simulink model "classification_model_1"  (R2018b)
settings: Solver=daessc  StartTime=0.0  StopTime=1  RelTol=1e-3
libraries: powerlib x7, powerlib_meascontrol x2
settings Model: Creator=Edagotti Pavankumar  LastModifiedBy=Edagotti Pavankumar
settings SolverCC: ZeroCrossAlgorithm=Adaptive
settings DebuggingCC: IgnoredZcDiagnostic=none

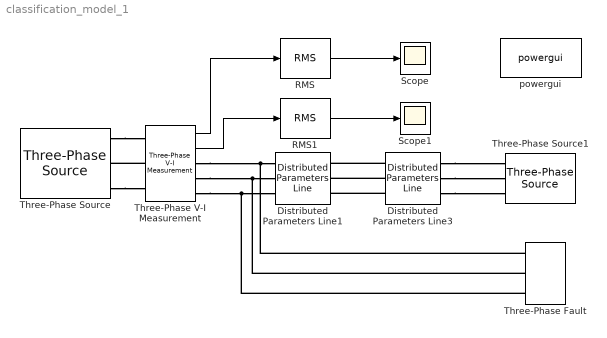
== system classification_model_1 ==
  Distributed Parameters Line1 : powerlib/Elements/Distributed Parameters Line  Phases=3  Frequency=50  Resistance=[0.0238 0.3885]  Inductance=[0.0009509508 0.0032508989]  Capacitance=[12.74e-9 7.751e-9]  Length=50  x1=[2.03029205726985e-09 272935.130000171 272935.130000166;314.159265358979 314.159265358979 314.159265358979;-1.05771318215586 0.434584098775176 -1.13621222801972]  x2=[2.17628988513287e-09 274142.447000751 274142.447000746;314.159265358979 314.159265358979 314.159265358979;-1.04287975057277 0.434398876325849 -1.13639745046905]  x3=[5.79526815658465e-12 1012.46010166729 1012.46010166727;314.159265358979 314.159265358979 314.159265358979;-1.58211710677278 0.326179290986126 -1.24461703580876]  x4=[8.43304661848584e-13 1012.22505654136 1012.22505654134;314.159265358979 314.159265358979 314.159265358979;-1.72619955217939 0.488614155737012 -1.08218217105788]  x5=0.000282770783497871  V1=[2.03e-09 2.729e+05 2.729e+05;314.2 314.2 314.2;-1.058 0.4346 -1.136]  V2=[2.176e-09 2.741e+05 2.741e+05;314.2 314.2 314.2;-1.043 0.4344 -1.136]  I1=[5.795e-12 1012 1012;314.2 314.2 314.2;-1.582 0.3262 -1.245]  I2=[8.433e-13 1012 1012;314.2 314.2 314.2;-1.726 0.4886 -1.082]  nHarmo=1  Measurements=None
      settings: SourceProductName=Simscape Power Systems
  Distributed Parameters Line3 : powerlib/Elements/Distributed Parameters Line  Phases=3  Frequency=50  Resistance=[0.0238 0.3885]  Inductance=[0.0009509508 0.0032508989]  Capacitance=[12.74e-9 7.751e-9]  Length=50  x1=[2.03029205726985e-09 272935.130000171 272935.130000166;314.159265358979 314.159265358979 314.159265358979;-1.05771318215586 0.434584098775176 -1.13621222801972]  x2=[2.17628988513287e-09 274142.447000751 274142.447000746;314.159265358979 314.159265358979 314.159265358979;-1.04287975057277 0.434398876325849 -1.13639745046905]  x3=[5.79526815658465e-12 1012.46010166729 1012.46010166727;314.159265358979 314.159265358979 314.159265358979;-1.58211710677278 0.326179290986126 -1.24461703580876]  x4=[8.43304661848584e-13 1012.22505654136 1012.22505654134;314.159265358979 314.159265358979 314.159265358979;-1.72619955217939 0.488614155737012 -1.08218217105788]  x5=0.000282770783497871  V1=[2.03e-09 2.729e+05 2.729e+05;314.2 314.2 314.2;-1.058 0.4346 -1.136]  V2=[2.176e-09 2.741e+05 2.741e+05;314.2 314.2 314.2;-1.043 0.4344 -1.136]  I1=[5.795e-12 1012 1012;314.2 314.2 314.2;-1.582 0.3262 -1.245]  I2=[8.433e-13 1012 1012;314.2 314.2 314.2;-1.726 0.4886 -1.082]  nHarmo=1  Measurements=None
      settings: SourceProductName=Simscape Power Systems
  RMS : powerlib_meascontrol/Measurements/RMS  TrueRMS=on  Freq=50  RMSInit=0  Ts=0
  RMS1 : powerlib_meascontrol/Measurements/RMS  TrueRMS=on  Freq=50  RMSInit=0  Ts=0
  Scope : Scope
  Scope1 : Scope
  Three-Phase V-I Measurement : powerlib/Measurements/Three-Phase V-I Measurement  VoltageMeasurement=phase-to-ground  SetLabelV=off  LabelV=Vabc  Vpu=on  VpuLL=off  CurrentMeasurement=yes  SetLabelI=off  LabelI=Iabc  Ipu=on  Pbase=100e6  Vbase=220e3  OutputType=Complex  PhasorSimulation=off  PSBequivalent=0
  Three-Phase Fault : powerlib/Elements/Three-Phase Fault  InitialStates=0  FaultA=on  FaultB=on  FaultC=on  GroundFault=on  SwitchTimes=0.5  External=off  SwitchStatus=NaN  FaultResistance=0.001  GroundResistance=0.001  SnubberResistance=1e6  SnubberCapacitance=inf  Measurements=None
  Three-Phase Source : powerlib/Electrical Sources/Three-Phase Source  InternalConnection=Yg  VoltagePhases=off  Voltage=220e3  PhaseAngle=0  Voltage_phases=[25e3 25e3 25e3]/sqrt(3)  PhaseAngles_phases=[0 -120 +120]  Frequency=50  NonIdealSource=on  SpecifyImpedance=on  Resistance=0.8929  Inductance=16.58e-3  ShortCircuitLevel=100e6  BaseVoltage=220e3  XRratio=7  BusType=swing  Pref=10e3  Qref=0  Prefabc=[10e3, 10e3, 10e3]  Qrefabc=[0, 0, 0]  Qmin=-inf  Qmax=inf
  Three-Phase Source1 : powerlib/Electrical Sources/Three-Phase Source  InternalConnection=Yg  VoltagePhases=off  Voltage=220e3  PhaseAngle=0  Voltage_phases=[25e3 25e3 25e3]/sqrt(3)  PhaseAngles_phases=[0 -120 +120]  Frequency=50  NonIdealSource=on  SpecifyImpedance=on  Resistance=0.8929  Inductance=16.58e-3  ShortCircuitLevel=100e6  BaseVoltage=220e3  XRratio=7  BusType=swing  Pref=10e3  Qref=0  Prefabc=[10e3, 10e3, 10e3]  Qrefabc=[0, 0, 0]  Qmin=-inf  Qmax=inf
  powergui : powerlib/powergui  Priority=1  SimulationMode=Continuous  SampleTime=50e-10  frequency=60  Iterations=50  frequencyindice=50  Pbase=100e6  ErrMax=1e-4  UnitsV=kV  UnitsW=MW  buscounter=0  FunctionMessages=off  echomessages=off  EnableUseOfTLC=off  CurrentSourceSwitches=off  DisableSnubberDevices=off  DisableRonSwitches=off  DisableVfSwitches=off  DisplayEquations=off  SolverType=Tustin/Backward Euler (TBE)  Interpol=off  ExternalGateDelay=off  methode=off  Ts=100  x0status=blocks  SPID=off  SwTol=0  HookPort=off  RestoreLinks=warning  ResistiveCurrentMeasurement=off  Frange=[0:2:500]  Ylog=off  Xlog=on  ShowGrid=off  save=off  variable=ZData  structure=0  ZoomFFT=off  StartTime=0.0  cycles=1  DisplayStyle=1  fundamental=60  FreqAxis=off  MaxFrequency=1000  frequencyindicesteady=1  RmsSteady=2  display=off
  wires:
  Three-Phase V-I Measurement/1 -> RMS/1
  RMS/1 -> Scope/1
  RMS1/1 -> Scope1/1
  Three-Phase V-I Measurement/2 -> RMS1/1
  connections:
  Three-Phase V-I Measurement/LConn2 -- Three-Phase Source/RConn2
  Three-Phase Source/RConn1 -- Three-Phase V-I Measurement/LConn1
  Three-Phase Source/RConn3 -- Three-Phase V-I Measurement/LConn3
  Three-Phase V-I Measurement/RConn1 -- Three-Phase Fault/LConn1 -- Distributed Parameters Line1/LConn1
  Three-Phase V-I Measurement/RConn2 -- Three-Phase Fault/LConn2 -- Distributed Parameters Line1/LConn2
  Three-Phase V-I Measurement/RConn3 -- Three-Phase Fault/LConn3 -- Distributed Parameters Line1/LConn3
  Distributed Parameters Line3/RConn1 -- Three-Phase Source1/RConn1
  Distributed Parameters Line3/RConn2 -- Three-Phase Source1/RConn2
  Distributed Parameters Line3/RConn3 -- Three-Phase Source1/RConn3
  Distributed Parameters Line3/LConn1 -- Distributed Parameters Line1/RConn1
  Distributed Parameters Line3/LConn2 -- Distributed Parameters Line1/RConn2
  Distributed Parameters Line3/LConn3 -- Distributed Parameters Line1/RConn3
